simulink model "SF051A_SnsrOffsLrng"  (R2013b)
settings: Solver=FixedStepDiscrete  SolverMode=SingleTasking  StartTime=0.0  StopTime=1  FixedStep=0.002  RelTol=1e-3
values from neighbouring files (symbols this model uses):
  ARCHGLBPRM_10MILLISEC_SEC_F32 = DataDict.Constant    [SF051A_SnsrOffsLrng_DataDict.m]
  ARCHGLBPRM_2MILLISEC_SEC_F32 = DataDict.Constant    [SF051A_SnsrOffsLrng_DataDict.m]
  ARCHGLBPRM_2PI_ULS_F32 = DataDict.Constant    [SF051A_SnsrOffsLrng_DataDict.m]
  ARCHGLBPRM_FLOATZEROTHD_ULS_F32 = DataDict.Constant    [SF051A_SnsrOffsLrng_DataDict.m]
  ARCHGLBPRM_PIOVER180_ULS_F32 = DataDict.Constant    [SF051A_SnsrOffsLrng_DataDict.m]
  CNV100MICROSECTOSEC_SECPERCNT_F32 = DataDict.Constant    [SF051A_SnsrOffsLrng_DataDict.m]
  COVRAMTRXNIT_ULS_F32 = DataDict.Constant    [SF051A_SnsrOffsLrng_DataDict.m]
  HWAGHILIM_HWDEG_F32 = DataDict.Constant    [SF051A_SnsrOffsLrng_DataDict.m]
  HWAUTHYTHD_ULS_F32 = DataDict.Constant    [SF051A_SnsrOffsLrng_DataDict.m]
  HWTQLRNGSTSLRND_CNT_U08 = DataDict.Constant    [SF051A_SnsrOffsLrng_DataDict.m]
  HWTQLRNGSTSNEGOFFS_CNT_U08 = DataDict.Constant    [SF051A_SnsrOffsLrng_DataDict.m]
  HWTQLRNGSTSNOTLRND_CNT_U08 = DataDict.Constant    [SF051A_SnsrOffsLrng_DataDict.m]
  HWTQLRNGSTSPOSOFFS_CNT_U08 = DataDict.Constant    [SF051A_SnsrOffsLrng_DataDict.m]
  HWTQLRNGSTSZEROOFFS_CNT_U08 = DataDict.Constant    [SF051A_SnsrOffsLrng_DataDict.m]
  IDYMTRX_ULS_F32 = DataDict.Constant    [SF051A_SnsrOffsLrng_DataDict.m]
  IVS10MS_ULSPERSEC_F32 = DataDict.Constant    [SF051A_SnsrOffsLrng_DataDict.m]
  LRNGFILTICON_ULS_F32 = DataDict.Constant    [SF051A_SnsrOffsLrng_DataDict.m]
  ONE_ULS_F32 = DataDict.Constant    [SF051A_SnsrOffsLrng_DataDict.m]
  SnsrOffsLrnd = DataDict.NVM    [SF051A_SnsrOffsLrng_DataDict.m]
  SnsrOffsLrngFctEna = DataDict.Calibration    [SF051A_SnsrOffsLrng_DataDict.m]
  SnsrOffsLrngHwAgLrngDrvgDstThd = DataDict.Calibration    [SF051A_SnsrOffsLrng_DataDict.m]
  SnsrOffsLrngHwAgLrngEna = DataDict.Calibration    [SF051A_SnsrOffsLrng_DataDict.m]
  SnsrOffsLrngHwAgLrngHwVelThd = DataDict.Calibration    [SF051A_SnsrOffsLrng_DataDict.m]
  SnsrOffsLrngHwAgLrngSysTqThd = DataDict.Calibration    [SF051A_SnsrOffsLrng_DataDict.m]
  SnsrOffsLrngHwAgLrngSysTqThdMed = DataDict.Calibration    [SF051A_SnsrOffsLrng_DataDict.m]
  SnsrOffsLrngHwAgLrngSysTqThdTrustd = DataDict.Calibration    [SF051A_SnsrOffsLrng_DataDict.m]
  SnsrOffsLrngHwAgLrngSysTqThdWide = DataDict.Calibration    [SF051A_SnsrOffsLrng_DataDict.m]
  SnsrOffsLrngHwAgLrngTi = DataDict.Calibration    [SF051A_SnsrOffsLrng_DataDict.m]
  SnsrOffsLrngHwAgLrngVehSpdThd = DataDict.Calibration    [SF051A_SnsrOffsLrng_DataDict.m]
  SnsrOffsLrngHwAgLrngYawOffsDbnd = DataDict.Calibration    [SF051A_SnsrOffsLrng_DataDict.m]
  SnsrOffsLrngHwAgLrngYawRateThd = DataDict.Calibration    [SF051A_SnsrOffsLrng_DataDict.m]
  SnsrOffsLrngHwAgOffsLim = DataDict.Calibration    [SF051A_SnsrOffsLrng_DataDict.m]
  SnsrOffsLrngHwTqLrngEna = DataDict.Calibration    [SF051A_SnsrOffsLrng_DataDict.m]
  SnsrOffsLrngHwTqLrngEnaTiThd = DataDict.Calibration    [SF051A_SnsrOffsLrng_DataDict.m]
  SnsrOffsLrngHwTqLrngHwAgDbnd = DataDict.Calibration    [SF051A_SnsrOffsLrng_DataDict.m]
  SnsrOffsLrngHwTqLrngHwAgThd = DataDict.Calibration    [SF051A_SnsrOffsLrng_DataDict.m]
  SnsrOffsLrngHwTqLrngHwTqThd = DataDict.Calibration    [SF051A_SnsrOffsLrng_DataDict.m]
  SnsrOffsLrngHwTqLrngHwTqZeroOffsThd = DataDict.Calibration    [SF051A_SnsrOffsLrng_DataDict.m]
  SnsrOffsLrngHwTqLrngHwVelThd = DataDict.Calibration    [SF051A_SnsrOffsLrng_DataDict.m]
  SnsrOffsLrngHwTqLrngMeasTi = DataDict.Calibration    [SF051A_SnsrOffsLrng_DataDict.m]
  SnsrOffsLrngHwTqLrngMeasTiScar = DataDict.Calibration    [SF051A_SnsrOffsLrng_DataDict.m]
  SnsrOffsLrngHwTqLrngSampleImbThd1 = DataDict.Calibration    [SF051A_SnsrOffsLrng_DataDict.m]
  SnsrOffsLrngHwTqLrngSampleImbThd2 = DataDict.Calibration    [SF051A_SnsrOffsLrng_DataDict.m]
  SnsrOffsLrngHwTqLrngSampleThd1 = DataDict.Calibration    [SF051A_SnsrOffsLrng_DataDict.m]
  SnsrOffsLrngHwTqLrngSampleThd2 = DataDict.Calibration    [SF051A_SnsrOffsLrng_DataDict.m]
  SnsrOffsLrngHwTqLrngTiWghtCoeff = DataDict.Calibration    [SF051A_SnsrOffsLrng_DataDict.m]
  SnsrOffsLrngHwTqLrngVehSpdThd = DataDict.Calibration    [SF051A_SnsrOffsLrng_DataDict.m]
  SnsrOffsLrngHwTqOffsLim = DataDict.Calibration    [SF051A_SnsrOffsLrng_DataDict.m]
  SnsrOffsLrngSampleCntForHwTqLrngRst = DataDict.Calibration    [SF051A_SnsrOffsLrng_DataDict.m]
  SnsrOffsLrngTqInpDetnPwrEstimnThd = DataDict.Calibration    [SF051A_SnsrOffsLrng_DataDict.m]
  SnsrOffsLrngTqInpDetnSinGenrAmp = DataDict.Calibration    [SF051A_SnsrOffsLrng_DataDict.m]
  SnsrOffsLrngTqInpDetnSinGenrFrq = DataDict.Calibration    [SF051A_SnsrOffsLrng_DataDict.m]
  SnsrOffsLrngTqInpDetnStg1FilGain = DataDict.Calibration    [SF051A_SnsrOffsLrng_DataDict.m]
  SnsrOffsLrngTqInpDetnStg1WinSize = DataDict.Calibration    [SF051A_SnsrOffsLrng_DataDict.m]
  SnsrOffsLrngTqInpDetnStg2FilGainCen = DataDict.Calibration    [SF051A_SnsrOffsLrng_DataDict.m]
  SnsrOffsLrngTqInpDetnStg2FilGainDwn = DataDict.Calibration    [SF051A_SnsrOffsLrng_DataDict.m]
  SnsrOffsLrngTqInpDetnStg2FilGainUp = DataDict.Calibration    [SF051A_SnsrOffsLrng_DataDict.m]
  SnsrOffsLrngTqInpDetnStg2WinSize = DataDict.Calibration    [SF051A_SnsrOffsLrng_DataDict.m]
  SnsrOffsLrngYawLrngEna = DataDict.Calibration    [SF051A_SnsrOffsLrng_DataDict.m]
  SnsrOffsLrngYawLrngHwAgThd = DataDict.Calibration    [SF051A_SnsrOffsLrng_DataDict.m]
  SnsrOffsLrngYawLrngTi = DataDict.Calibration    [SF051A_SnsrOffsLrng_DataDict.m]
  SnsrOffsLrngYawLrngYawAThd = DataDict.Calibration    [SF051A_SnsrOffsLrng_DataDict.m]
  SnsrOffsLrngYawOffsFrshTiThd = DataDict.Calibration    [SF051A_SnsrOffsLrng_DataDict.m]
  SnsrOffsLrngYawRateOffsLim = DataDict.Calibration    [SF051A_SnsrOffsLrng_DataDict.m]
  SPDCNVN_MTRPERSECPERKPH_F32 = DataDict.Constant    [SF051A_SnsrOffsLrng_DataDict.m]
  SysGlbPrmSysTqRat = DataDict.ImprtdCal    [SF051A_SnsrOffsLrng_DataDict.m]
  TISTEP10MS_MINS_F32 = DataDict.Constant    [SF051A_SnsrOffsLrng_DataDict.m]
  TQINPDETNLOGGAIN_ULS_F32 = DataDict.Constant    [SF051A_SnsrOffsLrng_DataDict.m]
  YAWELPDTIHILIM_MINS_F32 = DataDict.Constant    [SF051A_SnsrOffsLrng_DataDict.m]
  YAWRATENOISE_VEHDEGPERSEC_F32 = DataDict.Constant    [SF051A_SnsrOffsLrng_DataDict.m]
  ZERO_ULS_F32 = DataDict.Constant    [SF051A_SnsrOffsLrng_DataDict.m]
  ZEROVECT_ULS_F32 = DataDict.Constant    [SF051A_SnsrOffsLrng_DataDict.m]
undefined symbols (not defined in the file or in its folder): NvmGetErrSts1
libraries: Fil x34, NxtrLim x20, FixdToFloat x17, FloatToFixd x16, simulink x12, NxtrAbslt x12, NxtrNvM x8, NxtrMath x3
(part 6 of 12)

== system SF051A_SnsrOffsLrng/SnsrOffsLrng/SnsrOffsLrngPer1/Learning/ForgettingFactor ==
  SampleCntTot : Inport  RequirementInfo="{'linktype_rmi_doors' '0000babd (/E-STEER Core/SubSystem Specifications/Application Functions/SF051A Sensor Offset Learning)' '#SF051A_243' 'true' 'REQ:  SF051A_243' '' } %GIDa_3a0dab8d_8899_4510_9d33_ef745ce09e6f"
  Constant1 : Constant  RequirementInfo="{'linktype_rmi_doors' '0000babd (/E-STEER Core/SubSystem Specifications/Application Functions/SF051A Sensor Offset Learning)' '#SF051A_243' 'true' 'REQ:  SF051A_243' '' } %GIDa_21d51c87_7466_4d2f_9d56_8aff611e59ee"  Value=SnsrOffsLrngSampleCntForHwTqLrngRst  OutDataTypeStr=uint16
      settings: AttributesFormatString=%<OutDataTypeStr>
  Data Type Conversion : DataTypeConversion  RequirementInfo="{'linktype_rmi_doors' '0000babd (/E-STEER Core/SubSystem Specifications/Application Functions/SF051A Sensor Offset Learning)' '#SF051A_243' 'true' 'REQ:  SF051A_243' '' } %GIDa_34adf385_e0dc_4431_ad93_b255baa8cd9d"  OutDataTypeStr=uint16
  If : If  RequirementInfo="{'linktype_rmi_doors' '0000babd (/E-STEER Core/SubSystem Specifications/Application Functions/SF051A Sensor Offset Learning)' '#SF051A_243' 'true' 'REQ:  SF051A_243' '' } %GIDa_00ffddbc_2a9f_416d_92ac_8237a6566e70"  IfExpression=u1  ShowElse=off
  Relational Operator1 : RelationalOperator  RequirementInfo="{'linktype_rmi_doors' '0000babd (/E-STEER Core/SubSystem Specifications/Application Functions/SF051A Sensor Offset Learning)' '#SF051A_243' 'true' 'REQ:  SF051A_243' '' } %GIDa_95506176_73f4_4ba9_b5c7_f4ff23f708dc"  Operator=>  OutDataTypeStr=boolean
  ResetHwTqLrng : Subsystem  RequirementInfo="{'linktype_rmi_doors' '0000babd (/E-STEER Core/SubSystem Specifications/Application Functions/SF051A Sensor Offset Learning)' '#SF051A_243' 'true' 'REQ:  SF051A_243' '' } %GIDa_ec203b45_d0a1_4c9b_964d_3dc0fb0c2020"  TreatAsAtomicUnit=on
  Subsystem5 : Subsystem  Description=|  mask(Copyright Information){none=on}
      | Copyright info block.                                               
      |                                                                     
      | Place copyright information at the top of every subsystem in design.
      mask prompts: none "No parameters"
      mask help: Place copyright information at the top of every subsystem in design.
      mask Display:
      | NxtrConf = 'Nexteer Confidential';
      | 
      | sys = bdroot; %handle for the current model ("system")
      | first = get_param(sys,'Created');
      | first = first(end-3:end);  %year is last four digits
      | 
      | last = get_param(sys,'LastModifiedDate');
      | if isempty(last)
      |     last = datestr(now,'yyyy');
      | else
      |     last = last(end-3:end);
      | end
      | 
      | if strcmp(first,last)
      |     fprintf('%s -- Copyright %s Nexteer',NxtrConf,first)
      | else
      |     fprintf('%s -- %s%s- %s Nexteer',NxtrConf,char(169),first,last)
      | end
  wires:
  Constant1/1 -> Relational Operator1/2
  Relational Operator1/1 -> If/1
  SampleCntTot/1 -> Data Type Conversion/1
  If/1 -> ResetHwTqLrng/Action
  Data Type Conversion/1 -> Relational Operator1/1

== system SF051A_SnsrOffsLrng/SnsrOffsLrng/SnsrOffsLrngPer1/Learning/HwPos vs HwTrq Model ==
  note: X2
  note: X1
  note: This block prepares the independent variable for the linear regression --> Y = A1*X1 + A2*X2+ B
      | Where: X1 = sin(HwAg)   nad     X2 = cos(HwAg)
  note: Convert to 3-element array.
  note: The considered mathematical model HwTq vs HwAg follows:
      |                    Y = A*sin(X + Phi) + B
      | Where:
      | -. X = HwAg
      | -. Y = HwTq
      | -. A is the HwTq reading when Tq_Off=0Nm, Phi=0Deg and HwAg=90°
      | -. Phi = HwAg_Offset
      | -. B = HwTq_Offset
      |
      | That model can also be written as:
      |                Y = A1*sin(X) + A2*cos(X) + B
      | Where: A = sqrt(A1^2+A2^2)   and   sin(Phi) = A2/A
      |
      | The RLSE estimates the parameters A1, A2 and B.
  HwAgMeasd : Inport  OutDataTypeStr=single
  Cos_f32 : NxtrMath/Cos_f32  SFunctionSpec=single y1 = Cos_f32(single u1)
      settings: AttributesFormatString=%<MaskType>
  Mux : Mux  Inputs=3
  Row vector : Reshape  OutputDimensionality=Row vector (2-D)  OutputDimensions=[1,3]
  Sin_f32 : NxtrMath/Sin_f32  SFunctionSpec=single y1 = Sin_f32(single u1)
      settings: AttributesFormatString=%<MaskType>
  Subsystem5 : Subsystem  Description=|  mask(Copyright Information){none=on}
      | Copyright info block.                                               
      |                                                                     
      | Place copyright information at the top of every subsystem in design.
      mask prompts: none "No parameters"
      mask help: Place copyright information at the top of every subsystem in design.
      mask Display:
      | NxtrConf = 'Nexteer Confidential';
      | 
      | sys = bdroot; %handle for the current model ("system")
      | first = get_param(sys,'Created');
      | first = first(end-3:end);  %year is last four digits
      | 
      | last = get_param(sys,'LastModifiedDate');
      | if isempty(last)
      |     last = datestr(now,'yyyy');
      | else
      |     last = last(end-3:end);
      | end
      | 
      | if strcmp(first,last)
      |     fprintf('%s -- Copyright %s Nexteer',NxtrConf,first)
      | else
      |     fprintf('%s -- %s%s- %s Nexteer',NxtrConf,char(169),first,last)
      | end
  X0 : Constant  Value=ONE_ULS_F32  OutDataTypeStr=single
      settings: AttributesFormatString=%<OutDataTypeStr>
  constant : Constant  Value=ARCHGLBPRM_PIOVER180_ULS_F32  OutDataTypeStr=single
  deg2rad : Product  Inputs=**  OutDataTypeStr=single
  XAry : Outport
  wires:
  deg2rad/1 -> Sin_f32/1, Cos_f32/1
  constant/1 -> deg2rad/2
  HwAgMeasd/1 -> deg2rad/1
  Row vector/1 -> XAry/1  "TqMdlXAry"
  Mux/1 -> Row vector/1
  X0/1 -> Mux/1
  Cos_f32/1 -> Mux/3  "CosHwAg_HwRadpS_T_f32"
  Sin_f32/1 -> Mux/2  "SinHwAg_HwRadpS_T_f32"

== system SF051A_SnsrOffsLrng/SnsrOffsLrng/SnsrOffsLrngPer1/Learning/Recursive Least Square Regression ==
  note: Note for Coder:
      | In Matlab, a mattrix [3x2] has 3 rows and 2 columns.
      | This notation will be followed inside these blocks  -->
  XAry : Inport
  HwTqMeasd : Inport  Port=2
  Calculate Covariance Matrix : Subsystem
  Calculate K Vector : Subsystem
  Subsystem5 : Subsystem  Description=|  mask(Copyright Information){none=on}
      | Copyright info block.                                               
      |                                                                     
      | Place copyright information at the top of every subsystem in design.
      mask prompts: none "No parameters"
      mask help: Place copyright information at the top of every subsystem in design.
      mask Display:
      | NxtrConf = 'Nexteer Confidential';
      | 
      | sys = bdroot; %handle for the current model ("system")
      | first = get_param(sys,'Created');
      | first = first(end-3:end);  %year is last four digits
      | 
      | last = get_param(sys,'LastModifiedDate');
      | if isempty(last)
      |     last = datestr(now,'yyyy');
      | else
      |     last = last(end-3:end);
      | end
      | 
      | if strcmp(first,last)
      |     fprintf('%s -- Copyright %s Nexteer',NxtrConf,first)
      | else
      |     fprintf('%s -- %s%s- %s Nexteer',NxtrConf,char(169),first,last)
      | end
  Update beta_k : Subsystem
  HwTqOffsEstimd : Outport
  A2 : Outport  Port=2
  wires:
  [X_k] -> Update beta_k/1(XAry)
  XAry/1 -> Calculate K Vector/1(XAry), [X_k]
  Update beta_k/1(HwTqOffsEstimd) -> HwTqOffsEstimd/1
  [X_k] -> Calculate Covariance Matrix/1(XAry)
  HwTqMeasd/1 -> Update beta_k/3(HwTqMeasd)
  Update beta_k/2(A2) -> A2/1
  Calculate K Vector/1(KVect) -> Update beta_k/2(KVect), Calculate Covariance Matrix/2(KVect)

== system SF051A_SnsrOffsLrng/SnsrOffsLrng/SnsrOffsLrngPer1/Learning/Subsystem5 ==

== system SF051A_SnsrOffsLrng/SnsrOffsLrng/SnsrOffsLrngPer1/Learning/Update_NvmRam ==
  HwTqDriftEstimnOnCentr : Inport
  Action Port : ActionPort  ActionType=then
  Constant3 : Constant  RequirementInfo="{'linktype_rmi_doors' '0000babd (/E-STEER Core/SubSystem Specifications/Application Functions/SF051A Sensor Offset Learning)' '#SF051A_190' 'true' 'REQ:  SF051A_190' '' } %GIDa_6dc44b8d_9f3d_43c8_80fa_fbe50c8cea83"  Value=SnsrOffsLrngHwTqOffsLim  OutDataTypeStr=single
  FloatToFixd_s16_f32 : FloatToFixd/FloatToFixd_s16_f32  Param1=12
  LimDyn_f32 : NxtrLim/LimDyn_f32  RequirementInfo="{'linktype_rmi_doors' '0000babd (/E-STEER Core/SubSystem Specifications/Application Functions/SF051A Sensor Offset Learning)' '#SF051A_190' 'true' 'REQ:  SF051A_190' '' } %GIDa_a95859b7_a762_4c8d_bd03_84d163434d71"
  NvmRam : DataStoreWrite  DataStoreName=SnsrOffsLrnd  DataStoreElements=SnsrOffsLrnd.HwTqOffs
  Subsystem5 : Subsystem  Description=|  mask(Copyright Information){none=on}
      | Copyright info block.                                               
      |                                                                     
      | Place copyright information at the top of every subsystem in design.
      mask prompts: none "No parameters"
      mask help: Place copyright information at the top of every subsystem in design.
      mask Display:
      | NxtrConf = 'Nexteer Confidential';
      | 
      | sys = bdroot; %handle for the current model ("system")
      | first = get_param(sys,'Created');
      | first = first(end-3:end);  %year is last four digits
      | 
      | last = get_param(sys,'LastModifiedDate');
      | if isempty(last)
      |     last = datestr(now,'yyyy');
      | else
      |     last = last(end-3:end);
      | end
      | 
      | if strcmp(first,last)
      |     fprintf('%s -- Copyright %s Nexteer',NxtrConf,first)
      | else
      |     fprintf('%s -- %s%s- %s Nexteer',NxtrConf,char(169),first,last)
      | end
  Unary Minus : UnaryMinus  RequirementInfo="{'linktype_rmi_doors' '0000babd (/E-STEER Core/SubSystem Specifications/Application Functions/SF051A Sensor Offset Learning)' '#SF051A_190' 'true' 'REQ:  SF051A_190' '' } %GIDa_a7123fff_4a4e_4e7a_bbb1_3e64357493ac"
  wires:
  HwTqDriftEstimnOnCentr/1 -> LimDyn_f32/1
  LimDyn_f32/1 -> FloatToFixd_s16_f32/1
  FloatToFixd_s16_f32/1 -> NvmRam/1
  Unary Minus/1 -> LimDyn_f32/2
  Constant3/1 -> LimDyn_f32/3, Unary Minus/1

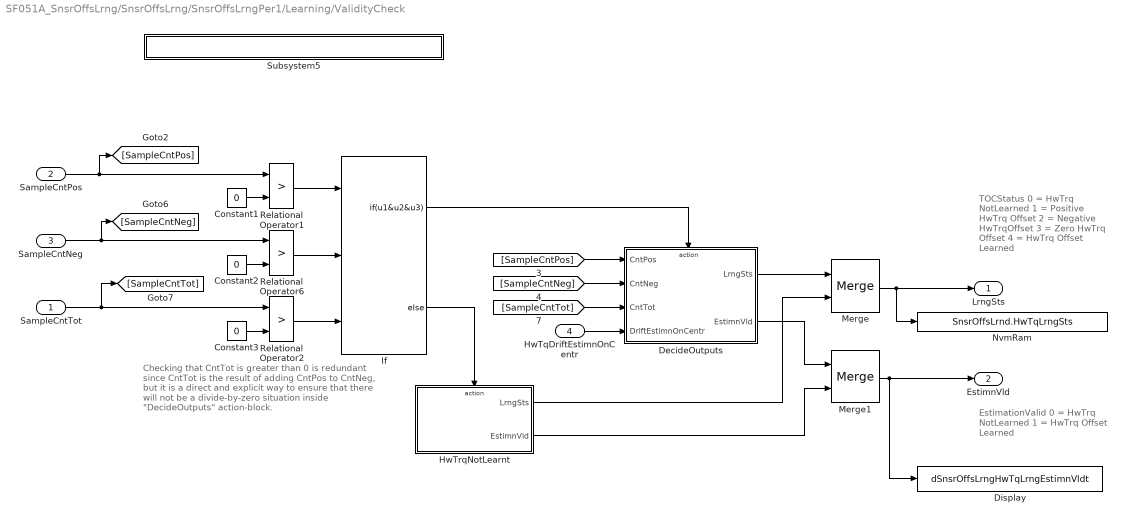
== system SF051A_SnsrOffsLrng/SnsrOffsLrng/SnsrOffsLrngPer1/Learning/ValidityCheck ==
  note: Checking that CntTot is greater than 0 is
      | redundant since CntTot is the result of adding
      | CntPos to CntNeg, but it is a direct and explicit
      | way to ensure that there will not be a divide-by-zero
      | situation inside "DecideOutputs" action-block.
  note: EstimationValid
      | 0 = HwTrq NotLearned
      | 1 = HwTrq Offset Learned
  note: TOCStatus
      | 0 = HwTrq NotLearned
      | 1 = Positive HwTrq Offset
      | 2 = Negative HwTrqOffset
      | 3 = Zero HwTrq Offset
      | 4 = HwTrq Offset Learned
  SampleCntTot : Inport
  SampleCntPos : Inport  Port=2
  SampleCntNeg : Inport  Port=3
  HwTqDriftEstimnOnCentr : Inport  Port=4
  Constant1 : Constant  Value=0  OutDataTypeStr=uint16
      settings: AttributesFormatString=%<OutDataTypeStr>
  Constant2 : Constant  Value=0  OutDataTypeStr=uint16
      settings: AttributesFormatString=%<OutDataTypeStr>
  Constant3 : Constant  Value=0  OutDataTypeStr=uint16
      settings: AttributesFormatString=%<OutDataTypeStr>
  DecideOutputs : Subsystem
  Display : DataStoreWrite  DataStoreName=dSnsrOffsLrngHwTqLrngEstimnVldt
  HwTrqNotLearnt : Subsystem  TreatAsAtomicUnit=on
  If : If  NumInputs=3  IfExpression=u1&u2&u3
  Merge : Merge
  Merge1 : Merge
  NvmRam : DataStoreWrite  DataStoreName=SnsrOffsLrnd  DataStoreElements=SnsrOffsLrnd.HwTqLrngSts
  Relational Operator1 : RelationalOperator  Operator=>  OutDataTypeStr=boolean
  Relational Operator2 : RelationalOperator  Operator=>  OutDataTypeStr=boolean
  Relational Operator6 : RelationalOperator  Operator=>  OutDataTypeStr=boolean
  Subsystem5 : Subsystem  Description=|  mask(Copyright Information){none=on}
      | Copyright info block.                                               
      |                                                                     
      | Place copyright information at the top of every subsystem in design.
      mask prompts: none "No parameters"
      mask help: Place copyright information at the top of every subsystem in design.
      mask Display:
      | NxtrConf = 'Nexteer Confidential';
      | 
      | sys = bdroot; %handle for the current model ("system")
      | first = get_param(sys,'Created');
      | first = first(end-3:end);  %year is last four digits
      | 
      | last = get_param(sys,'LastModifiedDate');
      | if isempty(last)
      |     last = datestr(now,'yyyy');
      | else
      |     last = last(end-3:end);
      | end
      | 
      | if strcmp(first,last)
      |     fprintf('%s -- Copyright %s Nexteer',NxtrConf,first)
      | else
      |     fprintf('%s -- %s%s- %s Nexteer',NxtrConf,char(169),first,last)
      | end
  LrngSts : Outport
  EstimnVld : Outport  Port=2
  wires:
  SampleCntNeg/1 -> [SampleCntNeg], Relational Operator6/1
  Constant2/1 -> Relational Operator6/2
  SampleCntPos/1 -> [SampleCntPos], Relational Operator1/1
  Relational Operator1/1 -> If/1
  Relational Operator6/1 -> If/2
  Constant1/1 -> Relational Operator1/2
  Constant3/1 -> Relational Operator2/2
  Relational Operator2/1 -> If/3
  [SampleCntPos] -> DecideOutputs/1(CntPos)
  [SampleCntNeg] -> DecideOutputs/2(CntNeg)
  [SampleCntTot] -> DecideOutputs/3(CntTot)
  HwTqDriftEstimnOnCentr/1 -> DecideOutputs/4(DriftEstimnOnCentr)
  DecideOutputs/1(LrngSts) -> Merge/1
  DecideOutputs/2(EstimnVld) -> Merge1/1
  If/1 -> DecideOutputs/Action
  Merge/1 -> LrngSts/1, NvmRam/1
  Merge1/1 -> Display/1, EstimnVld/1
  If/2 -> HwTrqNotLearnt/Action
  HwTrqNotLearnt/1(LrngSts) -> Merge/2
  HwTrqNotLearnt/2(EstimnVld) -> Merge1/2
  SampleCntTot/1 -> [SampleCntTot], Relational Operator2/1

== system SF051A_SnsrOffsLrng/SnsrOffsLrng/SnsrOffsLrngPer1/Measurements_Grabber/False ==
  Action Port : ActionPort  ActionType=then
  Constant : Constant  Value=false  OutDataTypeStr=boolean
      settings: AttributesFormatString=%<OutDataTypeStr>
  Constant2 : Constant  Value=ZERO_ULS_F32  OutDataTypeStr=single
      settings: AttributesFormatString=%<OutDataTypeStr>
  Subsystem5 : Subsystem  Description=|  mask(Copyright Information){none=on}
      | Copyright info block.                                               
      |                                                                     
      | Place copyright information at the top of every subsystem in design.
      mask prompts: none "No parameters"
      mask help: Place copyright information at the top of every subsystem in design.
      mask Display:
      | NxtrConf = 'Nexteer Confidential';
      | 
      | sys = bdroot; %handle for the current model ("system")
      | first = get_param(sys,'Created');
      | first = first(end-3:end);  %year is last four digits
      | 
      | last = get_param(sys,'LastModifiedDate');
      | if isempty(last)
      |     last = datestr(now,'yyyy');
      | else
      |     last = last(end-3:end);
      | end
      | 
      | if strcmp(first,last)
      |     fprintf('%s -- Copyright %s Nexteer',NxtrConf,first)
      | else
      |     fprintf('%s -- %s%s- %s Nexteer',NxtrConf,char(169),first,last)
      | end
  HwTqLrngLrngEna : Outport
  HwTq : Outport  Port=2
  HwAg : Outport  Port=3
  wires:
  Constant/1 -> HwTqLrngLrngEna/1
  Constant2/1 -> HwAg/1, HwTq/1

== system SF051A_SnsrOffsLrng/SnsrOffsLrng/SnsrOffsLrngPer1/Measurements_Grabber/GetTiSpan100MicroSec32bit ==
  note: Subtract original reference time
  note: seconds
  note: microseconds
  note: counts
  note: Wrap-to-zero
  note: 1 count = 100 uSec
  note: Get current system time
  note: GetTiSpan100MicroSec32bit
  note: Created Aug 18, 2015
      | Modified Oct 21, 2015
      | Modified Oct 30, 2015
      | Kevin Derry
  RefTmr : Inport
  CopyRight2 : Subsystem  Description=|  mask(Copyright Information){none=on}
      | Copyright info block.                                               
      |                                                                     
      | Place copyright information at the top of every subsystem in design.
      mask prompts: none "No parameters"
      mask help: Place copyright information at the top of every subsystem in design.
      mask Display:
      | NxtrConf = 'Nexteer Confidential';
      | 
      | sys = bdroot; %handle for the current model ("system")
      | first = get_param(sys,'Created');
      | if(isempty(first))
      |     first = datestr(now,'yyyy');
      | else
      |     first = first(end-3:end);  %year is last four digits
      | end
      | 
      | last = get_param(sys,'LastModifiedDate');
      | if isempty(last)
      |     last = datestr(now,'yyyy');
      | else
      |     last = last(end-3:end);
      | end
      | 
      | if strcmp(first,last)
      |     fprintf('%s -- Copyright %s Nexteer',NxtrConf,first)
      | else
      |     fprintf('%s -- %s%s- %s Nexteer',NxtrConf,char(169),first,last)
      | end
  Count per uSec : Constant  Value=0.01
  Data Store Read1 : DataStoreRead  DataStoreName=SimnTi
  Data Type Conversion2 : DataTypeConversion  OutDataTypeStr=uint32
  Divide1 : Product  Inputs=**
  Divide2 : Product  Inputs=*/
  If : If  NumInputs=2  IfExpression=u1 >= u2
  Max Counts : Constant  Value=2^32-1
  Merge : Merge
  No wrapping : Subsystem  TreatAsAtomicUnit=on
  Product2 : Product
  Product3 : Product
  Rounding : Rounding
  Subtract3 : Sum  Inputs=+-
  Wrapping : Subsystem  TreatAsAtomicUnit=on
  uSec per Sec : Constant  Value=1000000
  TiSpan : Outport
  wires:
  Wrapping/1(Out1) -> Merge/2
  No wrapping/1(Out1) -> Merge/1
  If/2 -> Wrapping/Action
  If/1 -> No wrapping/Action
  Product3/1 -> Subtract3/2
  Subtract3/1 -> Data Type Conversion2/1
  Rounding/1 -> Product3/1
  Divide2/1 -> Rounding/1
  Max Counts/1 -> Divide2/2, Product3/2
  Divide1/1 -> Divide2/1, Subtract3/1
  Product2/1 -> Divide1/1
  Data Store Read1/1 -> Product2/1
  Count per uSec/1 -> Divide1/2
  uSec per Sec/1 -> Product2/2
  Merge/1 -> TiSpan/1
  RefTmr/1 -> If/2, No wrapping/2(ref), Wrapping/2(ref)
  Data Type Conversion2/1 -> If/1, No wrapping/1(new), Wrapping/1(new)

== system SF051A_SnsrOffsLrng/SnsrOffsLrng/SnsrOffsLrngPer1/Measurements_Grabber/Subsystem5 ==

== system SF051A_SnsrOffsLrng/SnsrOffsLrng/SnsrOffsLrngPer1/Measurements_Grabber/True_UpdateNVMRam ==
  note: Set the Grabber Timer Reference back to current time.
  HwTq_in : Inport
  HwAg_in : Inport  Port=2
  Action Port : ActionPort  ActionType=else
  Constant : Constant  RequirementInfo="{'linktype_rmi_doors' '0000babd (/E-STEER Core/SubSystem Specifications/Application Functions/SF051A Sensor Offset Learning)' '#SF051A_154' 'true' 'REQ:  SF051A_154' '' } %GIDa_348884a7_199b_420e_8b8f_aec7d8a42fd4"  Value=true  OutDataTypeStr=boolean
      settings: AttributesFormatString=%<OutDataTypeStr>
  Data Store Write : DataStoreWrite  DataStoreName=HwTqLrngMeasTmrRef
  FloatToFixd_s16_f32 : FloatToFixd/FloatToFixd_s16_f32  Param1=4
  GetRefTmr100MicroSec32bit : Subsystem
  NvmRam : DataStoreWrite  RequirementInfo={'linktype_rmi_doors' '0000babd (/E-STEER Core/SubSystem Specifications/Application Functions/SF051A Sensor Offset Learning)' '#SF051A_153' 'true' 'REQ: SF051A_153' '' } %GIDa_33126d3e_f2c5_434b_b28a_2b62a4ba3060  DataStoreName=SnsrOffsLrnd  DataStoreElements=SnsrOffsLrnd.HwTqLrngHwAgRef
  Subsystem5 : Subsystem  Description=|  mask(Copyright Information){none=on}
      | Copyright info block.                                               
      |                                                                     
      | Place copyright information at the top of every subsystem in design.
      mask prompts: none "No parameters"
      mask help: Place copyright information at the top of every subsystem in design.
      mask Display:
      | NxtrConf = 'Nexteer Confidential';
      | 
      | sys = bdroot; %handle for the current model ("system")
      | first = get_param(sys,'Created');
      | first = first(end-3:end);  %year is last four digits
      | 
      | last = get_param(sys,'LastModifiedDate');
      | if isempty(last)
      |     last = datestr(now,'yyyy');
      | else
      |     last = last(end-3:end);
      | end
      | 
      | if strcmp(first,last)
      |     fprintf('%s -- Copyright %s Nexteer',NxtrConf,first)
      | else
      |     fprintf('%s -- %s%s- %s Nexteer',NxtrConf,char(169),first,last)
      | end
  HwTqLrngLrngEna : Outport  RequirementInfo="{'linktype_rmi_doors' '0000babd (/E-STEER Core/SubSystem Specifications/Application Functions/SF051A Sensor Offset Learning)' '#SF051A_154' 'true' 'REQ:  SF051A_154' '' } %GIDa_4152f285_7238_40df_a9ce_ba8c043104c1"
  HwTq : Outport  Port=2
  HwAg : Outport  Port=3
  wires:
  Constant/1 -> HwTqLrngLrngEna/1
  HwAg_in/1 -> FloatToFixd_s16_f32/1, HwAg/1
  HwTq_in/1 -> HwTq/1
  GetRefTmr100MicroSec32bit/1(RefTmr) -> Data Store Write/1
  FloatToFixd_s16_f32/1 -> NvmRam/1

== system SF051A_SnsrOffsLrng/SnsrOffsLrng/SnsrOffsLrngPer1/SetFalse/Subsystem1 ==

== system SF051A_SnsrOffsLrng/SnsrOffsLrng/SnsrOffsLrngPer1/Zero_GrabberTimer/GetRefTmr100MicroSec32bit ==
  note: 1 count = 100 uSec
  note: seconds
  note: microseconds
  note: counts
  note: Wrap-to-zero
  note: GetRefTmr100MicroSec32bit
  note: Created Aug 18, 2015
      | Modified Oct 21, 2015
      | Modified Oct 30, 2015
      | Kevin Derry
  CopyRight2 : Subsystem  Description=|  mask(Copyright Information){none=on}
      | Copyright info block.                                               
      |                                                                     
      | Place copyright information at the top of every subsystem in design.
      mask prompts: none "No parameters"
      mask help: Place copyright information at the top of every subsystem in design.
      mask Display:
      | NxtrConf = 'Nexteer Confidential';
      | 
      | sys = bdroot; %handle for the current model ("system")
      | first = get_param(sys,'Created');
      | if(isempty(first))
      |     first = datestr(now,'yyyy');
      | else
      |     first = first(end-3:end);  %year is last four digits
      | end
      | 
      | last = get_param(sys,'LastModifiedDate');
      | if isempty(last)
      |     last = datestr(now,'yyyy');
      | else
      |     last = last(end-3:end);
      | end
      | 
      | if strcmp(first,last)
      |     fprintf('%s -- Copyright %s Nexteer',NxtrConf,first)
      | else
      |     fprintf('%s -- %s%s- %s Nexteer',NxtrConf,char(169),first,last)
      | end
  Count per uSec : Constant  Value=0.01
  Data Store Read1 : DataStoreRead  DataStoreName=SimnTi
  Data Type Conversion1 : DataTypeConversion  OutDataTypeStr=uint32
  Divide1 : Product  Inputs=**
  Divide2 : Product  Inputs=*/
  Max Counts : Constant  Value=2^32-1
  Product1 : Product
  Product2 : Product
  Rounding : Rounding
  Subtract1 : Sum  Inputs=+-
  uSec per Sec : Constant  Value=1000000
  RefTmr : Outport
  wires:
  Product2/1 -> Subtract1/2
  Subtract1/1 -> Data Type Conversion1/1
  Rounding/1 -> Product2/1
  Divide2/1 -> Rounding/1
  Max Counts/1 -> Divide2/2, Product2/2
  Divide1/1 -> Divide2/1, Subtract1/1
  Product1/1 -> Divide1/1
  Count per uSec/1 -> Divide1/2
  uSec per Sec/1 -> Product1/2
  Data Type Conversion1/1 -> RefTmr/1
  Data Store Read1/1 -> Product1/1

== system SF051A_SnsrOffsLrng/SnsrOffsLrng/SnsrOffsLrngPer1/Zero_GrabberTimer/Subsystem5 ==

== system SF051A_SnsrOffsLrng/SnsrOffsLrng/SnsrOffsLrngPer2/Do nothing/Subsystem5 ==

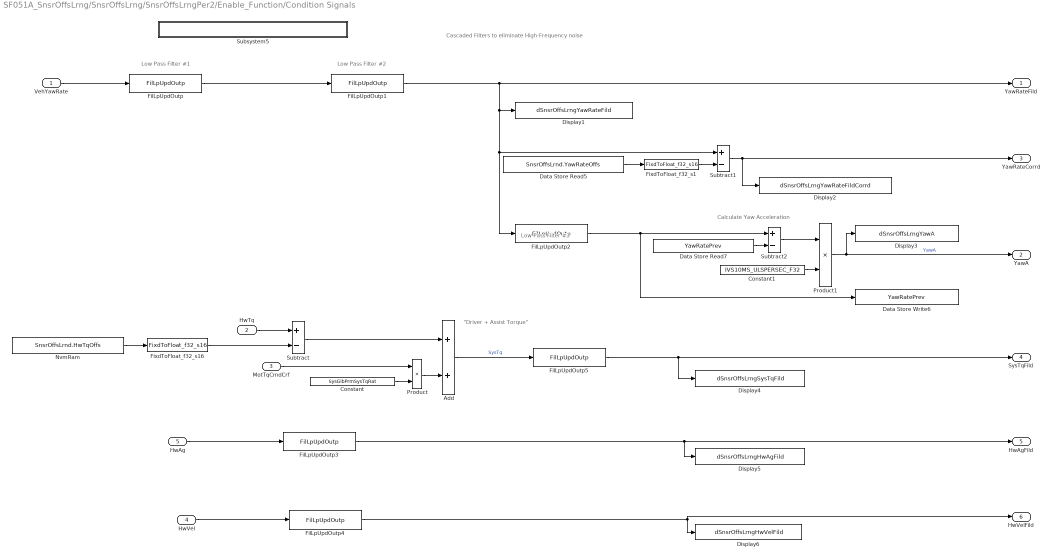
== system SF051A_SnsrOffsLrng/SnsrOffsLrng/SnsrOffsLrngPer2/Enable_Function/Condition Signals ==
  note: Calculate Yaw Acceleration
  note: Low Pass Filter #1
  note: Cascaded Filters to eliminate High-Frequency noise
  note: Low Pass Filter #2
  note: "Driver + Assist Torque"
  note: Low Pass Filter #3
  VehYawRate : Inport
  HwTq : Inport  RequirementInfo="{'linktype_rmi_doors' '0000babd (/E-STEER Core/SubSystem Specifications/Application Functions/SF051A Sensor Offset Learning)' '#SF051A_88' 'true' 'REQ:  SF051A_88' '' } %GIDa_cb0b5578_d931_4b15_8fb5_23406b09174e"  Port=2
  MotTqCmdCrf : Inport  RequirementInfo="{'linktype_rmi_doors' '0000babd (/E-STEER Core/SubSystem Specifications/Application Functions/SF051A Sensor Offset Learning)' '#SF051A_87' 'true' 'REQ:  SF051A_87' '' } %GIDa_6e162c2c_edb1_407c_9856_d4fb5c13668b"  Port=3
  HwVel : Inport  Port=4
  HwAg : Inport  Port=5
  Add : Sum  RequirementInfo="{'linktype_rmi_doors' '0000babd (/E-STEER Core/SubSystem Specifications/Application Functions/SF051A Sensor Offset Learning)' '#SF051A_87' 'true' 'REQ:  SF051A_87' '' } %GIDa_ae37b931_f532_4a31_8fdb_8a3b99cf0b70"
  Constant : Constant  RequirementInfo="{'linktype_rmi_doors' '0000babd (/E-STEER Core/SubSystem Specifications/Application Functions/SF051A Sensor Offset Learning)' '#SF051A_87' 'true' 'REQ:  SF051A_87' '' } %GIDa_19f7d8cf_06b3_41bf_b52b_b35be25960ea"  Value=SysGlbPrmSysTqRat
  Constant1 : Constant  RequirementInfo="{'linktype_rmi_doors' '0000babd (/E-STEER Core/SubSystem Specifications/Application Functions/SF051A Sensor Offset Learning)' '#SF051A_89' 'true' 'REQ:  SF051A_89' '' } %GIDa_346656a3_816f_4164_b776_9fdc6d4ed815"  Value=IVS10MS_ULSPERSEC_F32  OutDataTypeStr=single
  Data Store Read5 : DataStoreRead  RequirementInfo="{'linktype_rmi_doors' '0000babd (/E-STEER Core/SubSystem Specifications/Application Functions/SF051A Sensor Offset Learning)' '#SF051A_29' 'true' 'REQ:  SF051A_29' '' } %GIDa_fe5ea230_6dba_49b3_a98a_1e7dfb304a5e"  DataStoreName=SnsrOffsLrnd  DataStoreElements=SnsrOffsLrnd.YawRateOffs
  Data Store Read7 : DataStoreRead  RequirementInfo="{'linktype_rmi_doors' '0000babd (/E-STEER Core/SubSystem Specifications/Application Functions/SF051A Sensor Offset Learning)' '#SF051A_89' 'true' 'REQ:  SF051A_89' '' } %GIDa_851ad77d_6e53_4d8f_a6a0_8bfa0b715fb5"  Priority=1  DataStoreName=YawRatePrev
      settings: AttributesFormatString=priority: %<Priority>
  Data Store Write6 : DataStoreWrite  Priority=2  DataStoreName=YawRatePrev
      settings: AttributesFormatString=priority: %<Priority>
  Display1 : DataStoreWrite  DataStoreName=dSnsrOffsLrngYawRateFild
  Display2 : DataStoreWrite  DataStoreName=dSnsrOffsLrngYawRateFildCorrd
  Display3 : DataStoreWrite  DataStoreName=dSnsrOffsLrngYawA
  Display4 : DataStoreWrite  DataStoreName=dSnsrOffsLrngSysTqFild
  Display5 : DataStoreWrite  DataStoreName=dSnsrOffsLrngHwAgFild
  Display6 : DataStoreWrite  DataStoreName=dSnsrOffsLrngHwVelFild
  FilLpUpdOutp : Fil/FilLpUpdOutp  RequirementInfo={'linktype_rmi_doors' '0000babd (/E-STEER Core/SubSystem Specifications/Application Functions/SF051A Sensor Offset Learning)' '#SF051A_28' 'true' 'REQ: SF051A_28' '' } %GIDa_8a84e711_3ffa_4571_bf4b_e7f85249d077  StVar=YawCdngFil1
      settings: AttributesFormatString=StVar: %<StVar>
  FilLpUpdOutp1 : Fil/FilLpUpdOutp  RequirementInfo={'linktype_rmi_doors' '0000babd (/E-STEER Core/SubSystem Specifications/Application Functions/SF051A Sensor Offset Learning)' '#SF051A_28' 'true' 'REQ: SF051A_28' '' } %GIDa_c79bec69_8b23_4153_99a8_6f46e3270235  StVar=YawCdngFil2
      settings: AttributesFormatString=StVar: %<StVar>
  FilLpUpdOutp2 : Fil/FilLpUpdOutp  StVar=YawACdngFil
      settings: AttributesFormatString=StVar: %<StVar>
  FilLpUpdOutp3 : Fil/FilLpUpdOutp  RequirementInfo="{'linktype_rmi_doors' '0000babd (/E-STEER Core/SubSystem Specifications/Application Functions/SF051A Sensor Offset Learning)' '#SF051A_28' 'true' 'REQ:  SF051A_28' '' } %GIDa_cea2d234_d78b_493c_8f76_fa1ba10d1cf3"  StVar=HwAgCdngFil
      settings: AttributesFormatString=StVar: %<StVar>
  FilLpUpdOutp4 : Fil/FilLpUpdOutp  RequirementInfo="{'linktype_rmi_doors' '0000babd (/E-STEER Core/SubSystem Specifications/Application Functions/SF051A Sensor Offset Learning)' '#SF051A_28' 'true' 'REQ:  SF051A_28' '' } %GIDa_c5648a7c_47c7_487c_beaa_905359562805"  StVar=HwVelCdngFil
      settings: AttributesFormatString=StVar: %<StVar>
  FilLpUpdOutp5 : Fil/FilLpUpdOutp  RequirementInfo="{'linktype_rmi_doors' '0000babd (/E-STEER Core/SubSystem Specifications/Application Functions/SF051A Sensor Offset Learning)' '#SF051A_28' 'true' 'REQ:  SF051A_28' '' } %GIDa_a435df6e_5d26_4266_822f_3dfbe8640535"  StVar=SysTqCdngFil
      settings: AttributesFormatString=StVar: %<StVar>
  FixdToFloat_f32_s1 : FixdToFloat/FixdToFloat_f32_s16  RequirementInfo="{'linktype_rmi_doors' '0000babd (/E-STEER Core/SubSystem Specifications/Application Functions/SF051A Sensor Offset Learning)' '#SF051A_29' 'true' 'REQ:  SF051A_29' '' } %GIDa_3d73e24e_fd42_443d_a6ec_262aa8637762"  Param1=9
  FixdToFloat_f32_s16 : FixdToFloat/FixdToFloat_f32_s16  RequirementInfo="{'linktype_rmi_doors' '0000babd (/E-STEER Core/SubSystem Specifications/Application Functions/SF051A Sensor Offset Learning)' '#SF051A_88' 'true' 'REQ:  SF051A_88' '' } %GIDa_748ccc23_09d4_473b_a4ee_8bbea57db921"  Param1=12
  NvmRam : DataStoreRead  RequirementInfo="{'linktype_rmi_doors' '0000babd (/E-STEER Core/SubSystem Specifications/Application Functions/SF051A Sensor Offset Learning)' '#SF051A_88' 'true' 'REQ:  SF051A_88' '' } %GIDa_4121cf44_6622_4a9b_8e6c_74768dd324f4"  DataStoreName=SnsrOffsLrnd  DataStoreElements=SnsrOffsLrnd.HwTqOffs
  Product : Product  RequirementInfo="{'linktype_rmi_doors' '0000babd (/E-STEER Core/SubSystem Specifications/Application Functions/SF051A Sensor Offset Learning)' '#SF051A_87' 'true' 'REQ:  SF051A_87' '' } %GIDa_e0b80c88_6c4b_4ba5_b309_b8f72dd11838"
  Product1 : Product  RequirementInfo="{'linktype_rmi_doors' '0000babd (/E-STEER Core/SubSystem Specifications/Application Functions/SF051A Sensor Offset Learning)' '#SF051A_89' 'true' 'REQ:  SF051A_89' '' } %GIDa_0d782124_913b_4f0a_847b_c237fe5371b9"
  Subsystem5 : Subsystem  Description=|  mask(Copyright Information){none=on}
      | Copyright info block.                                               
      |                                                                     
      | Place copyright information at the top of every subsystem in design.
      mask prompts: none "No parameters"
      mask help: Place copyright information at the top of every subsystem in design.
      mask Display:
      | NxtrConf = 'Nexteer Confidential';
      | 
      | sys = bdroot; %handle for the current model ("system")
      | first = get_param(sys,'Created');
      | first = first(end-3:end);  %year is last four digits
      | 
      | last = get_param(sys,'LastModifiedDate');
      | if isempty(last)
      |     last = datestr(now,'yyyy');
      | else
      |     last = last(end-3:end);
      | end
      | 
      | if strcmp(first,last)
      |     fprintf('%s -- Copyright %s Nexteer',NxtrConf,first)
      | else
      |     fprintf('%s -- %s%s- %s Nexteer',NxtrConf,char(169),first,last)
      | end
  Subtract : Sum  RequirementInfo="{'linktype_rmi_doors' '0000babd (/E-STEER Core/SubSystem Specifications/Application Functions/SF051A Sensor Offset Learning)' '#SF051A_88' 'true' 'REQ:  SF051A_88' '' ; 'linktype_rmi_doors' '0000babd (/E-STEER Core/SubSystem Specifications/Application Functions/SF051A Sensor Offset Learning)' '#SF051A_87' 'true' 'REQ:  SF051A_87' '' } %GIDa_99fe81ca_b737_406d_903a_82e012cba0fe"  Inputs=+-
  Subtract1 : Sum  RequirementInfo="{'linktype_rmi_doors' '0000babd (/E-STEER Core/SubSystem Specifications/Application Functions/SF051A Sensor Offset Learning)' '#SF051A_29' 'true' 'REQ:  SF051A_29' '' } %GIDa_5e83f16f_2d18_4316_802f_cef8993711a6"  Inputs=+-
  Subtract2 : Sum  RequirementInfo="{'linktype_rmi_doors' '0000babd (/E-STEER Core/SubSystem Specifications/Application Functions/SF051A Sensor Offset Learning)' '#SF051A_89' 'true' 'REQ:  SF051A_89' '' } %GIDa_c77efd6a_eb15_4122_9f5d_3e3beff93d42"  Inputs=+-
  YawRateFild : Outport
  YawA : Outport  Port=2
  YawRateCorrd : Outport  Port=3  OutDataTypeStr=single
  SysTqFild : Outport  Port=4
  HwAgFild : Outport  Port=5
  HwVelFild : Outport  Port=6
  wires:
  VehYawRate/1 -> FilLpUpdOutp/1
  FilLpUpdOutp1/1 -> Display1/1, FilLpUpdOutp2/1, Subtract1/1, YawRateFild/1
  HwTq/1 -> Subtract/1
  FixdToFloat_f32_s16/1 -> Subtract/2
  Subtract/1 -> Add/1
  MotTqCmdCrf/1 -> Product/1
  Product/1 -> Add/2
  Constant/1 -> Product/2
  HwAg/1 -> FilLpUpdOutp3/1
  FilLpUpdOutp3/1 -> Display5/1, HwAgFild/1
  Add/1 -> FilLpUpdOutp5/1  "SysTq"
  HwVel/1 -> FilLpUpdOutp4/1
  FilLpUpdOutp4/1 -> HwVelFild/1, Display6/1
  Data Store Read5/1 -> FixdToFloat_f32_s1/1
  Subtract1/1 -> Display2/1, YawRateCorrd/1
  FilLpUpdOutp2/1 -> Data Store Write6/1, Subtract2/1
  Subtract2/1 -> Product1/1
  Constant1/1 -> Product1/2
  Product1/1 -> Display3/1, YawA/1  "YawA"
  Data Store Read7/1 -> Subtract2/2
  NvmRam/1 -> FixdToFloat_f32_s16/1
  FixdToFloat_f32_s1/1 -> Subtract1/2
  FilLpUpdOutp/1 -> FilLpUpdOutp1/1
  FilLpUpdOutp5/1 -> Display4/1, SysTqFild/1

== system SF051A_SnsrOffsLrng/SnsrOffsLrng/SnsrOffsLrngPer2/Enable_Function/POC ==
  note: Reset HwTq learning if requested by Hierarch Manager routine.
  note: Learn HwAg Offset if contitions are appropriate
  YawRateCorrd : Inport  RequirementInfo="{'linktype_rmi_doors' '0000babd (/E-STEER Core/SubSystem Specifications/Application Functions/SF051A Sensor Offset Learning)' '#SF051A_131' 'true' 'REQ:  SF051A_131' '' } %GIDa_2241a612_69c9_42e1_bc9a_8143374c6a10"
  SysTqFild : Inport  RequirementInfo="{'linktype_rmi_doors' '0000babd (/E-STEER Core/SubSystem Specifications/Application Functions/SF051A Sensor Offset Learning)' '#SF051A_130' 'true' 'REQ:  SF051A_130' '' } %GIDa_8ac64dc8_efd4_4fea_8be1_3530061f71ef"  Port=2
  HwAgFild : Inport  RequirementInfo="{'linktype_rmi_doors' '0000babd (/E-STEER Core/SubSystem Specifications/Application Functions/SF051A Sensor Offset Learning)' '#SF051A_132' 'true' 'REQ:  SF051A_132' '' } %GIDa_f9032355_6dd8_4cb3_b45a_f22c4cf0875b"  Port=3
  HwVelFild : Inport  RequirementInfo="{'linktype_rmi_doors' '0000babd (/E-STEER Core/SubSystem Specifications/Application Functions/SF051A Sensor Offset Learning)' '#SF051A_129' 'true' 'REQ:  SF051A_129' '' } %GIDa_c6634e4e_7c1b_460a_a499_07b7e4fc4f6e"  Port=4
  HwAgLrngEna : Inport  Port=5  OutDataTypeStr=boolean
  VehSpd : Inport  RequirementInfo="{'linktype_rmi_doors' '0000babd (/E-STEER Core/SubSystem Specifications/Application Functions/SF051A Sensor Offset Learning)' '#SF051A_133' 'true' 'REQ:  SF051A_133' '' } %GIDa_d75244df_0bb9_4d68_80fb_b65b4be69888"  Port=6
  HwTqLrngSts : Inport  RequirementInfo="{'linktype_rmi_doors' '0000babd (/E-STEER Core/SubSystem Specifications/Application Functions/SF051A Sensor Offset Learning)' '#SF051A_128' 'true' 'REQ:  SF051A_128' '' } %GIDa_340de515_3a73_4d29_9413_69b747b6f805"  Port=7
  HwAgLrngRst : Inport  Port=8
  Do nothing : Subsystem  TreatAsAtomicUnit=on
  Do nothing1 : Subsystem  TreatAsAtomicUnit=on
  If : If  RequirementInfo="{'linktype_rmi_doors' '0000babd (/E-STEER Core/SubSystem Specifications/Application Functions/SF051A Sensor Offset Learning)' '#SF051A_124' 'true' 'REQ:  SF051A_124' '' } %GIDa_5a1c07af_5997_48cd_9c05_bf217e97f002"  NumInputs=2  IfExpression=u1 & u2
  If1 : If  IfExpression=u1
  Learn : Subsystem  RequirementInfo="{'linktype_rmi_doors' '0000babd (/E-STEER Core/SubSystem Specifications/Application Functions/SF051A Sensor Offset Learning)' '#SF051A_127' 'true' 'REQ:  SF051A_127' '' } %GIDa_6eb60759_6337_4052_a701_a1794125d7b8"  TreatAsAtomicUnit=on
  Learning Conditions : Subsystem  RequirementInfo="{'linktype_rmi_doors' '0000babd (/E-STEER Core/SubSystem Specifications/Application Functions/SF051A Sensor Offset Learning)' '#SF051A_126' 'true' 'REQ:  SF051A_126' '' } %GIDa_668521da_dfcc_45f6_9303_a91806d72581"
  Reset_HwAg_Learning : Subsystem  TreatAsAtomicUnit=on
  Subsystem5 : Subsystem  Description=|  mask(Copyright Information){none=on}
      | Copyright info block.                                               
      |                                                                     
      | Place copyright information at the top of every subsystem in design.
      mask prompts: none "No parameters"
      mask help: Place copyright information at the top of every subsystem in design.
      mask Display:
      | NxtrConf = 'Nexteer Confidential';
      | 
      | sys = bdroot; %handle for the current model ("system")
      | first = get_param(sys,'Created');
      | first = first(end-3:end);  %year is last four digits
      | 
      | last = get_param(sys,'LastModifiedDate');
      | if isempty(last)
      |     last = datestr(now,'yyyy');
      | else
      |     last = last(end-3:end);
      | end
      | 
      | if strcmp(first,last)
      |     fprintf('%s -- Copyright %s Nexteer',NxtrConf,first)
      | else
      |     fprintf('%s -- %s%s- %s Nexteer',NxtrConf,char(169),first,last)
      | end
  wires:
  VehSpd/1 -> Learning Conditions/1(VehSpd)
  HwAgFild/1 -> Learn/1(HwAgFild)
  HwVelFild/1 -> Learning Conditions/2(HwVelFild)
  YawRateCorrd/1 -> Learning Conditions/3(YawRateCorrd)
  HwAgLrngEna/1 -> If/1  "HwAgLrngEna"
  HwTqLrngSts/1 -> Learn/3(HwTqLrngSts)
  Learning Conditions/1(LrngCdnVld) -> If/2
  If/1 -> Learn/Action
  SysTqFild/1 -> Learn/2(SysTrqFild), Learning Conditions/4(SysTqFild)
  If/2 -> Do nothing/Action
  HwAgLrngRst/1 -> If1/1
  If1/1 -> Reset_HwAg_Learning/Action
  If1/2 -> Do nothing1/Action

== system SF051A_SnsrOffsLrng/SnsrOffsLrng/SnsrOffsLrngPer2/Enable_Function/SOaC_HierarchyManager ==
  YawRateOffsFrsh : Inport
  HwAgAuthy : Inport  Port=2
  VehSpdVld : Inport  Port=3
  VehYawRateVld : Inport  Port=4
  Constant : Constant  Value=HWAUTHYTHD_ULS_F32
  Logical Operator : Logic  AllPortsSameDT=off  OutDataTypeStr=boolean
  POCEnabler : Subsystem
  POCResetLogic : Subsystem
  Relational Operator : RelationalOperator  OutDataTypeStr=boolean
  Subsystem5 : Subsystem  Description=|  mask(Copyright Information){none=on}
      | Copyright info block.                                               
      |                                                                     
      | Place copyright information at the top of every subsystem in design.
      mask prompts: none "No parameters"
      mask help: Place copyright information at the top of every subsystem in design.
      mask Display:
      | NxtrConf = 'Nexteer Confidential';
      | 
      | sys = bdroot; %handle for the current model ("system")
      | first = get_param(sys,'Created');
      | first = first(end-3:end);  %year is last four digits
      | 
      | last = get_param(sys,'LastModifiedDate');
      | if isempty(last)
      |     last = datestr(now,'yyyy');
      | else
      |     last = last(end-3:end);
      | end
      | 
      | if strcmp(first,last)
      |     fprintf('%s -- Copyright %s Nexteer',NxtrConf,first)
      | else
      |     fprintf('%s -- %s%s- %s Nexteer',NxtrConf,char(169),first,last)
      | end
  YOCEnabler : Subsystem
  YawRateLrngEna : Outport
  HwAgLrngEna : Outport  Port=2
  HwAgLrngRst : Outport  Port=3
  wires:
  POCResetLogic/1(HwAgLrngRst) -> HwAgLrngRst/1
  POCEnabler/1(HwAgLrngEna) -> HwAgLrngEna/1
  YOCEnabler/1(YawRateLrngEna) -> YawRateLrngEna/1
  Relational Operator/1 -> Logical Operator/1
  VehSpdVld/1 -> Logical Operator/2
  VehYawRateVld/1 -> YOCEnabler/2(VehYawRateVld), POCEnabler/2(VehYawRateVld)
  HwAgAuthy/1 -> Relational Operator/1
  Logical Operator/1 -> YOCEnabler/1(CmnSigVld), [CmnSigVld]  "CmnSigVld"
  [CmnSigVld] -> POCEnabler/1(CmnSigVld)
  YawRateOffsFrsh/1 -> POCEnabler/3(YawRateOffsFrsh)
  Constant/1 -> Relational Operator/2

== system SF051A_SnsrOffsLrng/SnsrOffsLrng/SnsrOffsLrngPer2/Enable_Function/Subsystem5 ==
